simulink model "arducopter"  (R2021a)
settings: Solver=FixedStepAuto  StartTime=0.0  StopTime=sim.param.timeEnd  FixedStep=sim.param.dt  RelTol=1e-3
undefined symbols (not defined in the file or in its folder): DiscIntNeverNeededParam, sim
libraries: simulink x34, slident x4, vrlib x1
(part 2 of 8)

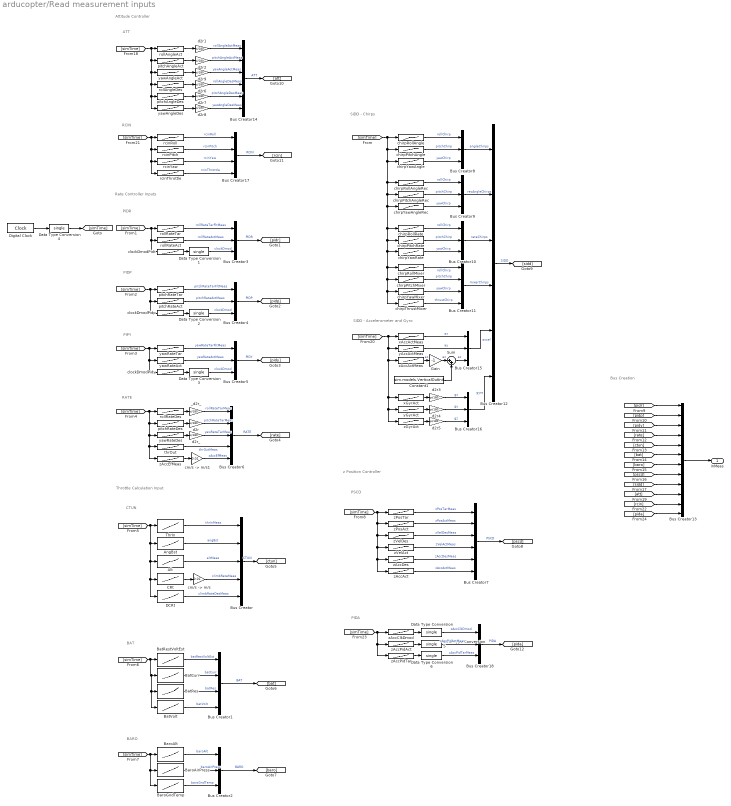
== system arducopter/Read measurement inputs ==
  note: PIDA
  note: Rate Controller Inputs
  note: SIDD - Chirps
  note: PIDR
  note: PIDP
  note: PIPY
  note: RATE
  note: CTUN
  note: BAT
  note: BARO
  note: Throttle Calculation Input
  note: PSCD
  note: z Position Controller
  note: Bus Creation
  note: ATT
  note: Attitude Controller
  note: SIDD - Accelerometer and Gyro
  note: RCIN
  Alt : Lookup_n-D  NumberOfTableDimensions=1  BreakpointsForDimension1=sim.signals.CTUN.Time  Table=sim.signals.CTUN.Alt  TableDataTypeStr=single  InternalRulePriority=Speed  OutDataTypeStr=Inherit: Inherit from 'Table data'  RndMeth=Simplest  InputSameDT=on
  AngBst : Lookup_n-D  NumberOfTableDimensions=1  BreakpointsForDimension1=sim.signals.CTUN.Time  Table=sim.signals.CTUN.AngBst  TableDataTypeStr=single  InternalRulePriority=Speed  OutDataTypeStr=Inherit: Inherit from 'Table data'  RndMeth=Simplest  InputSameDT=on
  BaroAirPress : Lookup_n-D  NumberOfTableDimensions=1  BreakpointsForDimension1=sim.signals.BARO.Time  Table=sim.signals.BARO.AirPress  TableDataTypeStr=Inherit: Inherit from 'Table data'  InternalRulePriority=Speed  OutDataTypeStr=Inherit: Inherit from 'Table data'  RndMeth=Simplest  InputSameDT=on
  BaroAlt : Lookup_n-D  NumberOfTableDimensions=1  BreakpointsForDimension1=sim.signals.BARO.Time  Table=sim.signals.BARO.Alt  TableDataTypeStr=Inherit: Inherit from 'Table data'  InternalRulePriority=Speed  OutDataTypeStr=Inherit: Inherit from 'Table data'  RndMeth=Simplest  InputSameDT=on
  BaroGndTemp : Lookup_n-D  NumberOfTableDimensions=1  BreakpointsForDimension1=sim.signals.BARO.Time  Table=sim.signals.BARO.GndTemp  TableDataTypeStr=Inherit: Inherit from 'Table data'  InternalRulePriority=Speed  OutDataTypeStr=Inherit: Inherit from 'Table data'  RndMeth=Simplest  InputSameDT=on
  BatCurr : Lookup_n-D  NumberOfTableDimensions=1  BreakpointsForDimension1=sim.signals.BAT.Time  Table=sim.signals.BAT.Curr  TableDataTypeStr=single  InternalRulePriority=Speed  OutDataTypeStr=Inherit: Inherit from 'Table data'  RndMeth=Simplest  InputSameDT=on
  BatRes : Lookup_n-D  NumberOfTableDimensions=1  BreakpointsForDimension1=sim.signals.BAT.Time  Table=sim.signals.BAT.Res  TableDataTypeStr=single  InternalRulePriority=Speed  OutDataTypeStr=Inherit: Inherit from 'Table data'  RndMeth=Simplest  InputSameDT=on
  BatRestVoltEst : Lookup_n-D  NumberOfTableDimensions=1  BreakpointsForDimension1=sim.signals.BAT.Time  Table=sim.signals.BAT.RestVoltEst  TableDataTypeStr=single  InternalRulePriority=Speed  OutDataTypeStr=Inherit: Inherit from 'Table data'  RndMeth=Simplest  InputSameDT=on
  BatVolt : Lookup_n-D  NumberOfTableDimensions=1  BreakpointsForDimension1=sim.signals.BAT.Time  Table=sim.signals.BAT.Volt  TableDataTypeStr=Inherit: Inherit from 'Table data'  InternalRulePriority=Speed  OutDataTypeStr=Inherit: Inherit from 'Table data'  RndMeth=Simplest  InputSameDT=on
  Bus Creator : BusCreator  Inputs=5
  Bus Creator1 : BusCreator  Inputs=4
  Bus Creator{2..5,8..10,15..16,18} (10 alike) : BusCreator  Inputs=3
  Bus Creator11 : BusCreator  Inputs=4
  Bus Creator12 : BusCreator  Inputs=6
  Bus Creator13 : BusCreator  Inputs=12
  Bus Creator14 : BusCreator  Inputs=6
  Bus Creator17 : BusCreator  Inputs=4
  Bus Creator6 : BusCreator  Inputs=5
  Bus Creator7 : BusCreator  Inputs=6
  CRt : Lookup_n-D  NumberOfTableDimensions=1  BreakpointsForDimension1=sim.signals.CTUN.Time  Table=sim.signals.CTUN.CRt  TableDataTypeStr=single  InternalRulePriority=Speed  OutDataTypeStr=Inherit: Inherit from 'Table data'  RndMeth=Simplest  InputSameDT=on
  Constant1 : Constant  Value=sim.models.VerticalOutInit
  DCRt : Lookup_n-D  NumberOfTableDimensions=1  BreakpointsForDimension1=sim.signals.CTUN.Time  Table=sim.signals.CTUN.DCRt  TableDataTypeStr=single  InternalRulePriority=Speed  OutDataTypeStr=Inherit: Inherit from 'Table data'  RndMeth=Simplest  InputSameDT=on
  Data Type Conversion{,1..6} (7 alike) : DataTypeConversion  OutDataTypeStr=single
  Digital Clock : DigitalClock  SampleTime=sim.param.dt
  Gain : Gain  Gain=-1
  Sum : Sum  Inputs=|++
  ThrIn : Lookup_n-D  NumberOfTableDimensions=1  BreakpointsForDimension1=sim.signals.CTUN.Time  Table=sim.signals.CTUN.ThrIn  TableDataTypeStr=single  InternalRulePriority=Speed  OutDataTypeStr=Inherit: Inherit from 'Table data'  RndMeth=Simplest  InputSameDT=on
  _d2r_ : Gain  Gain=pi/180
  chirpPitchAngle : Lookup_n-D  NumberOfTableDimensions=1  BreakpointsForDimension1=sim.signals.SIDD.Time{2}  Table=sim.signals.SIDD.Chirp{2}  TableDataTypeStr=Inherit: Inherit from 'Table data'  InternalRulePriority=Speed  OutDataTypeStr=Inherit: Inherit from 'Table data'  RndMeth=Simplest  InputSameDT=on
  chirpPitchAngleRec : Lookup_n-D  NumberOfTableDimensions=1  BreakpointsForDimension1=sim.signals.SIDD.Time{5}  Table=sim.signals.SIDD.Chirp{5}  TableDataTypeStr=Inherit: Inherit from 'Table data'  InternalRulePriority=Speed  OutDataTypeStr=Inherit: Inherit from 'Table data'  RndMeth=Simplest  InputSameDT=on
  chirpPitchMixer : Lookup_n-D  NumberOfTableDimensions=1  BreakpointsForDimension1=sim.signals.SIDD.Time{11}  Table=sim.signals.SIDD.Chirp{11}  TableDataTypeStr=Inherit: Inherit from 'Table data'  InternalRulePriority=Speed  OutDataTypeStr=Inherit: Inherit from 'Table data'  RndMeth=Simplest  InputSameDT=on
  chirpPitchRate : Lookup_n-D  NumberOfTableDimensions=1  BreakpointsForDimension1=sim.signals.SIDD.Time{8}  Table=sim.signals.SIDD.Chirp{8}  TableDataTypeStr=Inherit: Inherit from 'Table data'  InternalRulePriority=Speed  OutDataTypeStr=Inherit: Inherit from 'Table data'  RndMeth=Simplest  InputSameDT=on
  chirpRollAngle : Lookup_n-D  NumberOfTableDimensions=1  BreakpointsForDimension1=sim.signals.SIDD.Time{1}  Table=sim.signals.SIDD.Chirp{1}  TableDataTypeStr=Inherit: Inherit from 'Table data'  InternalRulePriority=Speed  OutDataTypeStr=Inherit: Inherit from 'Table data'  RndMeth=Simplest  InputSameDT=on
  chirpRollAngleRec : Lookup_n-D  NumberOfTableDimensions=1  BreakpointsForDimension1=sim.signals.SIDD.Time{4}  Table=sim.signals.SIDD.Chirp{4}  TableDataTypeStr=Inherit: Inherit from 'Table data'  InternalRulePriority=Speed  OutDataTypeStr=Inherit: Inherit from 'Table data'  RndMeth=Simplest  InputSameDT=on
  chirpRollMixer : Lookup_n-D  NumberOfTableDimensions=1  BreakpointsForDimension1=sim.signals.SIDD.Time{10}  Table=sim.signals.SIDD.Chirp{10}  TableDataTypeStr=Inherit: Inherit from 'Table data'  InternalRulePriority=Speed  OutDataTypeStr=Inherit: Inherit from 'Table data'  RndMeth=Simplest  InputSameDT=on
  chirpRollRate : Lookup_n-D  NumberOfTableDimensions=1  BreakpointsForDimension1=sim.signals.SIDD.Time{7}  Table=sim.signals.SIDD.Chirp{7}  TableDataTypeStr=Inherit: Inherit from 'Table data'  InternalRulePriority=Speed  OutDataTypeStr=Inherit: Inherit from 'Table data'  RndMeth=Simplest  InputSameDT=on
  chirpThrustMixer : Lookup_n-D  NumberOfTableDimensions=1  BreakpointsForDimension1=sim.signals.SIDD.Time{13}  Table=sim.signals.SIDD.Chirp{13}  TableDataTypeStr=Inherit: Inherit from 'Table data'  InternalRulePriority=Speed  OutDataTypeStr=Inherit: Inherit from 'Table data'  RndMeth=Simplest  InputSameDT=on
  chirpYawAngle : Lookup_n-D  NumberOfTableDimensions=1  BreakpointsForDimension1=sim.signals.SIDD.Time{3}  Table=sim.signals.SIDD.Chirp{3}  TableDataTypeStr=Inherit: Inherit from 'Table data'  InternalRulePriority=Speed  OutDataTypeStr=Inherit: Inherit from 'Table data'  RndMeth=Simplest  InputSameDT=on
  chirpYawAngleRec : Lookup_n-D  NumberOfTableDimensions=1  BreakpointsForDimension1=sim.signals.SIDD.Time{6}  Table=sim.signals.SIDD.Chirp{6}  TableDataTypeStr=Inherit: Inherit from 'Table data'  InternalRulePriority=Speed  OutDataTypeStr=Inherit: Inherit from 'Table data'  RndMeth=Simplest  InputSameDT=on
  chirpYawMixer : Lookup_n-D  NumberOfTableDimensions=1  BreakpointsForDimension1=sim.signals.SIDD.Time{12}  Table=sim.signals.SIDD.Chirp{12}  TableDataTypeStr=Inherit: Inherit from 'Table data'  InternalRulePriority=Speed  OutDataTypeStr=Inherit: Inherit from 'Table data'  RndMeth=Simplest  InputSameDT=on
  chirpYawRate : Lookup_n-D  NumberOfTableDimensions=1  BreakpointsForDimension1=sim.signals.SIDD.Time{9}  Table=sim.signals.SIDD.Chirp{9}  TableDataTypeStr=Inherit: Inherit from 'Table data'  InternalRulePriority=Speed  OutDataTypeStr=Inherit: Inherit from 'Table data'  RndMeth=Simplest  InputSameDT=on
  clockDmodPidp : Lookup_n-D  NumberOfTableDimensions=1  BreakpointsForDimension1=sim.signals.PIDP.Time  Table=sim.signals.PIDP.ClockDMod  InternalRulePriority=Speed  RndMeth=Simplest  InputSameDT=on
  clockDmodPidr : Lookup_n-D  NumberOfTableDimensions=1  BreakpointsForDimension1=sim.signals.PIDR.Time  Table=sim.signals.PIDR.ClockDMod  TableDataTypeStr=Inherit: Inherit from 'Table data'  InternalRulePriority=Speed  OutDataTypeStr=Inherit: Inherit from 'Table data'  RndMeth=Simplest  InputSameDT=on
  clockDmodPidy : Lookup_n-D  NumberOfTableDimensions=1  BreakpointsForDimension1=sim.signals.PIDY.Time  Table=sim.signals.PIDY.ClockDMod  InternalRulePriority=Speed  RndMeth=Simplest  InputSameDT=on
  "cm/s -> m/s" : Gain  Gain=0.01
  "cm/s -> m/s1" : Gain  Gain=0.01
  d2r{,1..9} (10 alike) : Gain  Gain=pi/180
  d2r_ : Gain  Gain=pi/180
  pitchAngleAct : Lookup_n-D  NumberOfTableDimensions=1  BreakpointsForDimension1=sim.signals.ATT.Time  Table=sim.signals.ATT.Pitch  TableDataTypeStr=Inherit: Inherit from 'Table data'  InternalRulePriority=Speed  OutDataTypeStr=Inherit: Inherit from 'Table data'  RndMeth=Simplest  InputSameDT=on
  pitchAngleDes : Lookup_n-D  NumberOfTableDimensions=1  BreakpointsForDimension1=sim.signals.ATT.Time  Table=sim.signals.ATT.DesPitch  TableDataTypeStr=Inherit: Inherit from 'Table data'  InternalRulePriority=Speed  OutDataTypeStr=Inherit: Inherit from 'Table data'  RndMeth=Simplest  InputSameDT=on
  pitchRateAct : Lookup_n-D  NumberOfTableDimensions=1  BreakpointsForDimension1=sim.signals.PIDP.Time  Table=sim.signals.PIDP.Act  TableDataTypeStr=Inherit: Inherit from 'Table data'  InternalRulePriority=Speed  OutDataTypeStr=Inherit: Inherit from 'Table data'  RndMeth=Simplest  InputSameDT=on
  pitchRateDes : Lookup_n-D  NumberOfTableDimensions=1  BreakpointsForDimension1=sim.signals.RATE.Time  Table=sim.signals.RATE.PDes  TableDataTypeStr=Inherit: Inherit from 'Table data'  InternalRulePriority=Speed  OutDataTypeStr=Inherit: Inherit from 'Table data'  RndMeth=Simplest  InputSameDT=on
  pitchRateTar : Lookup_n-D  NumberOfTableDimensions=1  BreakpointsForDimension1=sim.signals.PIDP.Time  Table=sim.signals.PIDP.Tar  TableDataTypeStr=Inherit: Inherit from 'Table data'  InternalRulePriority=Speed  OutDataTypeStr=Inherit: Inherit from 'Table data'  RndMeth=Simplest  InputSameDT=on
  rcinPitch : Lookup_n-D  NumberOfTableDimensions=1  BreakpointsForDimension1=sim.signals.RCIN.Time  Table=sim.signals.RCIN.PitchInput  InterpMethod=Linear Lagrange  ExtrapMethod=Clip  InternalRulePriority=Speed  OutDataTypeStr=Inherit: Inherit from 'Table data'  RndMeth=Simplest  InputSameDT=on
  rcinRoll : Lookup_n-D  NumberOfTableDimensions=1  BreakpointsForDimension1=sim.signals.RCIN.Time  Table=sim.signals.RCIN.RollInput  TableDataTypeStr=Inherit: Inherit from 'Table data'  ExtrapMethod=Clip  InternalRulePriority=Speed  OutDataTypeStr=Inherit: Inherit from 'Table data'  RndMeth=Simplest  InputSameDT=on
  rcinThrottle : Lookup_n-D  NumberOfTableDimensions=1  BreakpointsForDimension1=sim.signals.RCIN.Time  Table=sim.signals.RCIN.ThrottleInput  TableDataTypeStr=Inherit: Inherit from 'Table data'  ExtrapMethod=Clip  InternalRulePriority=Speed  OutDataTypeStr=Inherit: Inherit from 'Table data'  RndMeth=Simplest  InputSameDT=on
  rcinYaw : Lookup_n-D  NumberOfTableDimensions=1  BreakpointsForDimension1=sim.signals.RCIN.Time  Table=sim.signals.RCIN.YawInput  TableDataTypeStr=Inherit: Inherit from 'Table data'  ExtrapMethod=Clip  InternalRulePriority=Speed  OutDataTypeStr=Inherit: Inherit from 'Table data'  RndMeth=Simplest  InputSameDT=on
  rollAngleAct : Lookup_n-D  NumberOfTableDimensions=1  BreakpointsForDimension1=sim.signals.ATT.Time  Table=sim.signals.ATT.Roll  TableDataTypeStr=Inherit: Inherit from 'Table data'  InternalRulePriority=Speed  OutDataTypeStr=Inherit: Inherit from 'Table data'  RndMeth=Simplest  InputSameDT=on
  rollAngleDes : Lookup_n-D  NumberOfTableDimensions=1  BreakpointsForDimension1=sim.signals.ATT.Time  Table=sim.signals.ATT.DesRoll  TableDataTypeStr=Inherit: Inherit from 'Table data'  InternalRulePriority=Speed  OutDataTypeStr=Inherit: Inherit from 'Table data'  RndMeth=Simplest  InputSameDT=on
  rollRateAct : Lookup_n-D  NumberOfTableDimensions=1  BreakpointsForDimension1=sim.signals.PIDR.Time  Table=sim.signals.PIDR.Act  TableDataTypeStr=Inherit: Inherit from 'Table data'  InternalRulePriority=Speed  OutDataTypeStr=Inherit: Inherit from 'Table data'  RndMeth=Simplest  InputSameDT=on
  rollRateDes : Lookup_n-D  NumberOfTableDimensions=1  BreakpointsForDimension1=sim.signals.RATE.Time  Table=sim.signals.RATE.RDes  TableDataTypeStr=Inherit: Inherit from 'Table data'  InternalRulePriority=Speed  OutDataTypeStr=Inherit: Inherit from 'Table data'  RndMeth=Simplest  InputSameDT=on
  rollRateTar : Lookup_n-D  NumberOfTableDimensions=1  BreakpointsForDimension1=sim.signals.PIDR.Time  Table=sim.signals.PIDR.Tar  TableDataTypeStr=Inherit: Inherit from 'Table data'  InternalRulePriority=Speed  OutDataTypeStr=Inherit: Inherit from 'Table data'  RndMeth=Simplest  InputSameDT=on
  thrOut : Lookup_n-D  NumberOfTableDimensions=1  BreakpointsForDimension1=sim.signals.RATE.Time  Table=sim.signals.RATE.AOut  TableDataTypeStr=Inherit: Inherit from 'Table data'  InternalRulePriority=Speed  OutDataTypeStr=Inherit: Inherit from 'Table data'  RndMeth=Simplest  InputSameDT=on
  xAccActMeas : Lookup_n-D  NumberOfTableDimensions=1  BreakpointsForDimension1=sim.signals.SIDD.Time{1}  Table=sim.signals.SIDD.AccX  TableDataTypeStr=Inherit: Inherit from 'Table data'  InternalRulePriority=Speed  OutDataTypeStr=Inherit: Inherit from 'Table data'  RndMeth=Simplest  InputSameDT=on
  xGyrAct : Lookup_n-D  NumberOfTableDimensions=1  BreakpointsForDimension1=sim.signals.SIDD.Time{1}  Table=sim.signals.SIDD.GyrX  TableDataTypeStr=Inherit: Inherit from 'Table data'  InternalRulePriority=Speed  OutDataTypeStr=Inherit: Inherit from 'Table data'  RndMeth=Simplest  InputSameDT=on
  yAccActMeas : Lookup_n-D  NumberOfTableDimensions=1  BreakpointsForDimension1=sim.signals.SIDD.Time{1}  Table=sim.signals.SIDD.AccY  TableDataTypeStr=Inherit: Inherit from 'Table data'  InternalRulePriority=Speed  OutDataTypeStr=Inherit: Inherit from 'Table data'  RndMeth=Simplest  InputSameDT=on
  yGyrAct : Lookup_n-D  NumberOfTableDimensions=1  BreakpointsForDimension1=sim.signals.SIDD.Time{1}  Table=sim.signals.SIDD.GyrY  TableDataTypeStr=Inherit: Inherit from 'Table data'  InternalRulePriority=Speed  OutDataTypeStr=Inherit: Inherit from 'Table data'  RndMeth=Simplest  InputSameDT=on
  yawAngleAct : Lookup_n-D  NumberOfTableDimensions=1  BreakpointsForDimension1=sim.signals.ATT.Time  Table=sim.signals.ATT.Yaw  TableDataTypeStr=Inherit: Inherit from 'Table data'  InternalRulePriority=Speed  OutDataTypeStr=Inherit: Inherit from 'Table data'  RndMeth=Simplest  InputSameDT=on
  yawAngleDes : Lookup_n-D  NumberOfTableDimensions=1  BreakpointsForDimension1=sim.signals.ATT.Time  Table=sim.signals.ATT.DesYaw  TableDataTypeStr=Inherit: Inherit from 'Table data'  InternalRulePriority=Speed  OutDataTypeStr=Inherit: Inherit from 'Table data'  RndMeth=Simplest  InputSameDT=on
  yawRateAct : Lookup_n-D  NumberOfTableDimensions=1  BreakpointsForDimension1=sim.signals.PIDY.Time  Table=sim.signals.PIDY.Act  TableDataTypeStr=Inherit: Inherit from 'Table data'  InternalRulePriority=Speed  OutDataTypeStr=Inherit: Inherit from 'Table data'  RndMeth=Simplest  InputSameDT=on
  yawRateDes : Lookup_n-D  NumberOfTableDimensions=1  BreakpointsForDimension1=sim.signals.RATE.Time  Table=sim.signals.RATE.YDes  TableDataTypeStr=Inherit: Inherit from 'Table data'  InternalRulePriority=Speed  OutDataTypeStr=Inherit: Inherit from 'Table data'  RndMeth=Simplest  InputSameDT=on
  yawRateTar : Lookup_n-D  NumberOfTableDimensions=1  BreakpointsForDimension1=sim.signals.PIDY.Time  Table=sim.signals.PIDY.Tar  TableDataTypeStr=Inherit: Inherit from 'Table data'  InternalRulePriority=Speed  OutDataTypeStr=Inherit: Inherit from 'Table data'  RndMeth=Simplest  InputSameDT=on
  zAccAct : Lookup_n-D  NumberOfTableDimensions=1  BreakpointsForDimension1=sim.signals.PSCD.Time  Table=sim.signals.PSCD.zAccAct  TableDataTypeStr=single  InternalRulePriority=Speed  OutDataTypeStr=Inherit: Inherit from 'Table data'  RndMeth=Simplest  InputSameDT=on
  zAccActMeas : Lookup_n-D  NumberOfTableDimensions=1  BreakpointsForDimension1=sim.signals.SIDD.Time{1}  Table=sim.signals.SIDD.AccZ  TableDataTypeStr=Inherit: Inherit from 'Table data'  InternalRulePriority=Speed  OutDataTypeStr=Inherit: Inherit from 'Table data'  RndMeth=Simplest  InputSameDT=on
  zAccClkDmod : Lookup_n-D  NumberOfTableDimensions=1  BreakpointsForDimension1=sim.signals.PIDA.Time  Table=sim.signals.PIDA.ClockDMod  InternalRulePriority=Speed  RndMeth=Simplest  InputSameDT=on
  zAccDes : Lookup_n-D  NumberOfTableDimensions=1  BreakpointsForDimension1=sim.signals.PSCD.Time  Table=sim.signals.PSCD.zAccDes  TableDataTypeStr=single  InternalRulePriority=Speed  OutDataTypeStr=Inherit: Inherit from 'Table data'  RndMeth=Simplest  InputSameDT=on
  zAccEfMeas : Lookup_n-D  NumberOfTableDimensions=1  BreakpointsForDimension1=sim.signals.RATE.Time  Table=sim.signals.RATE.A  TableDataTypeStr=Inherit: Inherit from 'Table data'  InternalRulePriority=Speed  OutDataTypeStr=Inherit: Inherit from 'Table data'  RndMeth=Simplest  InputSameDT=on
  zAccPidAct : Lookup_n-D  NumberOfTableDimensions=1  BreakpointsForDimension1=sim.signals.PIDA.Time  Table=sim.signals.PIDA.Act  InternalRulePriority=Speed  RndMeth=Simplest  InputSameDT=on
  zAccPidTar : Lookup_n-D  NumberOfTableDimensions=1  BreakpointsForDimension1=sim.signals.PIDA.Time  Table=sim.signals.PIDA.Tar  InternalRulePriority=Speed  RndMeth=Simplest  InputSameDT=on
  zGyrAct : Lookup_n-D  NumberOfTableDimensions=1  BreakpointsForDimension1=sim.signals.SIDD.Time{1}  Table=sim.signals.SIDD.GyrZ  TableDataTypeStr=Inherit: Inherit from 'Table data'  InternalRulePriority=Speed  OutDataTypeStr=Inherit: Inherit from 'Table data'  RndMeth=Simplest  InputSameDT=on
  zPosAct : Lookup_n-D  NumberOfTableDimensions=1  BreakpointsForDimension1=sim.signals.PSCD.Time  Table=sim.signals.PSCD.zPosAct  TableDataTypeStr=single  InternalRulePriority=Speed  OutDataTypeStr=Inherit: Inherit from 'Table data'  RndMeth=Simplest  InputSameDT=on
  zPosTar : Lookup_n-D  NumberOfTableDimensions=1  BreakpointsForDimension1=sim.signals.PSCD.Time  Table=sim.signals.PSCD.zPosTar  TableDataTypeStr=single  InternalRulePriority=Speed  OutDataTypeStr=Inherit: Inherit from 'Table data'  RndMeth=Simplest  InputSameDT=on
  zVelAct : Lookup_n-D  NumberOfTableDimensions=1  BreakpointsForDimension1=sim.signals.PSCD.Time  Table=sim.signals.PSCD.zVelAct  TableDataTypeStr=Inherit: Inherit from 'Table data'  InternalRulePriority=Speed  OutDataTypeStr=single  RndMeth=Simplest  InputSameDT=on
  zVelDes : Lookup_n-D  NumberOfTableDimensions=1  BreakpointsForDimension1=sim.signals.PSCD.Time  Table=sim.signals.PSCD.zVelDes  TableDataTypeStr=single  InternalRulePriority=Speed  OutDataTypeStr=Inherit: Inherit from 'Table data'  RndMeth=Simplest  InputSameDT=on
  inMeas : Outport
  wires:
  Digital Clock/1 -> Data Type Conversion4/1
  [simTime] -> chirpThrustMixer/1, chirpYawMixer/1, chirpPitchMixer/1, chirpRollMixer/1, chirpYawRate/1, chirpPitchRate/1, chirpRollRate/1, chirpYawAngleRec/1, chirpPitchAngleRec/1, chirpRollAngleRec/1, chirpYawAngle/1, chirpPitchAngle/1, chirpRollAngle/1
  [simTime] -> clockDmodPidr/1, rollRateAct/1, rollRateTar/1
  [simTime] -> clockDmodPidp/1, pitchRateAct/1, pitchRateTar/1
  [simTime] -> yawRateAct/1, clockDmodPidy/1, yawRateTar/1
  [simTime] -> rollRateDes/1, zAccEfMeas/1, thrOut/1, yawRateDes/1, pitchRateDes/1
  ThrIn/1 -> Bus Creator/1  "thrInMeas"
  BaroAlt/1 -> Bus Creator2/1  "baroAlt"
  BaroAirPress/1 -> Bus Creator2/2  "baroAirPress"
  AngBst/1 -> Bus Creator/2  "angBst"
  BatCurr/1 -> Bus Creator1/2  "batCurr"
  BatVolt/1 -> Bus Creator1/4  "batVolt"
  BaroGndTemp/1 -> Bus Creator2/3  "baroGndTemp"
  BatRes/1 -> Bus Creator1/3  "batRes"
  BatRestVoltEst/1 -> Bus Creator1/1  "batRestVoltEst"
  [simTime] -> CRt/1, DCRt/1, Alt/1, AngBst/1, ThrIn/1
  [simTime] -> BatVolt/1, BatRes/1, BatCurr/1, BatRestVoltEst/1
  [simTime] -> BaroGndTemp/1, BaroAirPress/1, BaroAlt/1
  rollRateTar/1 -> Bus Creator3/1  "rollRateTarFltMeas"
  clockDmodPidr/1 -> Data Type Conversion1/1
  pitchRateTar/1 -> Bus Creator4/1  "pitchRateTarFltMeas"
  clockDmodPidp/1 -> Data Type Conversion2/1
  yawRateAct/1 -> Bus Creator5/2  "yawRateActMeas"
  yawRateTar/1 -> Bus Creator5/1  "yawRateTarFltMeas"
  clockDmodPidy/1 -> Data Type Conversion3/1
  pitchRateDes/1 -> d2r/1
  rollRateDes/1 -> _d2r_/1
  yawRateDes/1 -> d2r_/1
  d2r_/1 -> Bus Creator6/3  "yawRateTarMeas"
  Bus Creator3/1 -> [pidr]  "PIDR"
  Bus Creator4/1 -> [pidp]  "PIDP"
  Bus Creator5/1 -> [pidy]  "PIDY"
  Bus Creator6/1 -> [rate]  "RATE"
  Bus Creator/1 -> [ctun]  "CTUN"
  Bus Creator1/1 -> [bat]  "BAT"
  Bus Creator2/1 -> [baro]  "BARO"
  zPosAct/1 -> Bus Creator7/2  "zPosActMeas"
  zVelDes/1 -> Bus Creator7/3  "zVelDesMeas"
  zVelAct/1 -> Bus Creator7/4  "zVelActMeas"
  zAccAct/1 -> Bus Creator7/6  "zAccActMeas"
  zPosTar/1 -> Bus Creator7/1  "zPosTarMeas"
  zAccDes/1 -> Bus Creator7/5  "zAccDesMeas"
  [simTime] -> zPosAct/1, zAccAct/1, zAccDes/1, zVelAct/1, zVelDes/1, zPosTar/1
  Bus Creator7/1 -> [pscd]  "PSCD"
  Data Type Conversion1/1 -> Bus Creator3/3  "clockDmod"
  Data Type Conversion2/1 -> Bus Creator4/3  "clockDmod"
  Data Type Conversion3/1 -> Bus Creator5/3  "clockDmod"
  chirpPitchAngle/1 -> Bus Creator8/2  "pitchChirp"
  chirpRollAngle/1 -> Bus Creator8/1  "rollChirp"
  chirpYawAngle/1 -> Bus Creator8/3  "yawChirp"
  Bus Creator8/1 -> Bus Creator12/1  "angleChirps"
  chirpPitchAngleRec/1 -> Bus Creator9/2  "pitchChirp"
  chirpRollAngleRec/1 -> Bus Creator9/1  "rollChirp"
  chirpYawAngleRec/1 -> Bus Creator9/3  "yawChirp"
  Bus Creator9/1 -> Bus Creator12/2  "recAngleChirps"
  chirpPitchRate/1 -> Bus Creator10/2  "pitchChirp"
  chirpRollRate/1 -> Bus Creator10/1  "rollChirp"
  chirpYawRate/1 -> Bus Creator10/3  "yawChirp"
  Bus Creator10/1 -> Bus Creator12/3  "rateChirps"
  chirpRollMixer/1 -> Bus Creator11/1  "rollChirp"
  chirpPitchMixer/1 -> Bus Creator11/2  "pitchChirp"
  chirpYawMixer/1 -> Bus Creator11/3  "yawChirp"
  Bus Creator11/1 -> Bus Creator12/4  "mixerChirps"
  chirpThrustMixer/1 -> Bus Creator11/4  "thrustChirp"
  Bus Creator12/1 -> [sidd]  "SIDD"
  Bus Creator13/1 -> inMeas/1
  [pidr] -> Bus Creator13/1
  [pidp] -> Bus Creator13/2
  [pidy] -> Bus Creator13/3
  [rate] -> Bus Creator13/4
  [ctun] -> Bus Creator13/5
  [bat] -> Bus Creator13/6
  [baro] -> Bus Creator13/7
  [pscd] -> Bus Creator13/8
  [sidd] -> Bus Creator13/9
  Data Type Conversion4/1 -> [simTime]
  pitchRateAct/1 -> Bus Creator4/2  "pitchRateActMeas"
  _d2r_/1 -> Bus Creator6/1  "rollRateTarMeas"
  rollRateAct/1 -> Bus Creator3/2  "rollRateActMeas"
  d2r/1 -> Bus Creator6/2  "pitchRateTarMeas"
  d2r2/1 -> Bus Creator14/2  "pitchAngleActMeas"
  Bus Creator14/1 -> [att]  "ATT"
  d2r1/1 -> Bus Creator14/1  "rollAngleActMeas"
  [simTime] -> rollAngleAct/1, yawAngleAct/1, yawAngleDes/1, pitchAngleDes/1, rollAngleDes/1, pitchAngleAct/1
  [att] -> Bus Creator13/10
  [simTime] -> zGyrAct/1, yGyrAct/1, xGyrAct/1, zAccActMeas/1, yAccActMeas/1, xAccActMeas/1
  xAccActMeas/1 -> Bus Creator15/1  "ax"
  yAccActMeas/1 -> Bus Creator15/2  "ay"
  xGyrAct/1 -> d2r3/1
  yGyrAct/1 -> d2r4/1
  zGyrAct/1 -> d2r5/1
  Bus Creator15/1 -> Bus Creator12/5  "accel"
  Bus Creator16/1 -> Bus Creator12/6  "gyro"
  rollAngleAct/1 -> d2r1/1
  pitchAngleAct/1 -> d2r2/1
  d2r3/1 -> Bus Creator16/1  "gx"
  d2r4/1 -> Bus Creator16/2  "gy"
  d2r5/1 -> Bus Creator16/3  "gz"
  pitchAngleDes/1 -> d2r7/1
  rollAngleDes/1 -> d2r6/1
  d2r6/1 -> Bus Creator14/4  "rollAngleDesMeas"
  d2r7/1 -> Bus Creator14/5  "pitchAngleDesMeas"
  yawAngleDes/1 -> d2r8/1
  d2r8/1 -> Bus Creator14/6  "yawAngleDesMeas"
  yawAngleAct/1 -> d2r9/1
  d2r9/1 -> Bus Creator14/3  "yawAngleActMeas"
  rcinRoll/1 -> Bus Creator17/1  "rcinRoll"
  rcinPitch/1 -> Bus Creator17/2  "rcinPitch"
  rcinYaw/1 -> Bus Creator17/3  "rcinYaw"
  Bus Creator17/1 -> [rcin]  "RCIN"
  [rcin] -> Bus Creator13/11
  [simTime] -> rcinRoll/1, rcinThrottle/1, rcinYaw/1, rcinPitch/1
  thrOut/1 -> Bus Creator6/4  "thrOutMeas"
  zAccEfMeas/1 -> "cm/s -> m/s1"/1
  zAccActMeas/1 -> Gain/1  "az"
  Alt/1 -> Bus Creator/3  "altMeas"
  CRt/1 -> "cm/s -> m/s"/1
  "cm/s -> m/s"/1 -> Bus Creator/4  "climbRateMeas"
  Sum/1 -> Bus Creator15/3  "az"
  "cm/s -> m/s1"/1 -> Bus Creator6/5  "zAccEfMeas"
  Gain/1 -> Sum/1  "az"
  Constant1/1 -> Sum/2
  Data Type Conversion/1 -> Bus Creator18/1  "zAccClkDmod"
  zAccClkDmod/1 -> Data Type Conversion/1
  [simTime] -> zAccPidTar/1, zAccPidAct/1, zAccClkDmod/1
  zAccPidAct/1 -> Data Type Conversion5/1
  zAccPidTar/1 -> Data Type Conversion6/1
  Data Type Conversion5/1 -> Bus Creator18/2  "zAccPidActMeas"
  Data Type Conversion6/1 -> Bus Creator18/3  "zAccPidTarMeas"
  Bus Creator18/1 -> [pida]  "PIDA"
  [pida] -> Bus Creator13/12
  DCRt/1 -> Bus Creator/5  "climbRateDesMeas"
  rcinThrottle/1 -> Bus Creator17/4  "rcinThrottle"

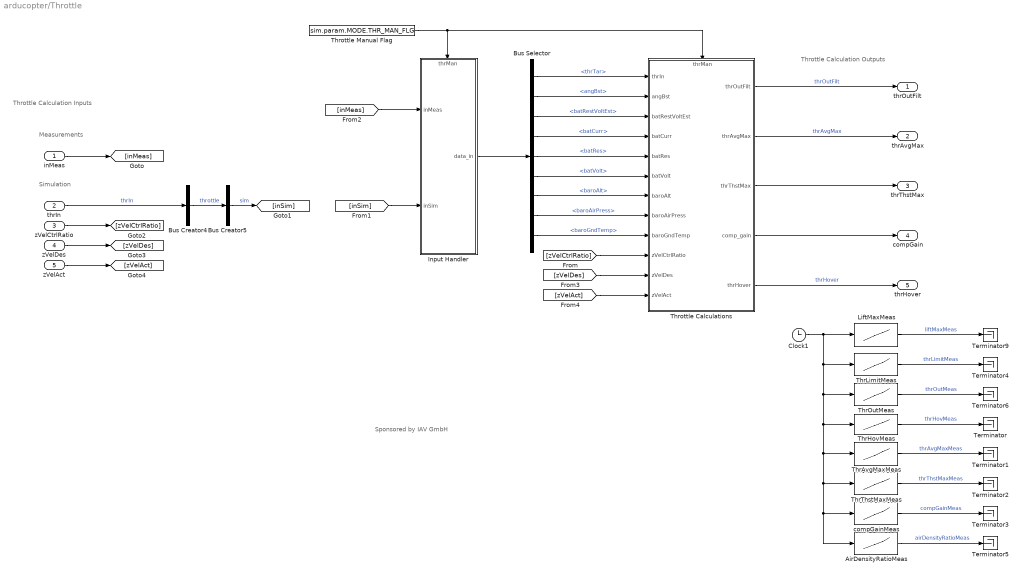
== system arducopter/Throttle ==
  note: Throttle Calculation Outputs
  note: Throttle Calculation Inputs
  note: Simulation
  note: Measurements
  note: Sponsored by IAV GmbH
  inMeas : Inport
  thrIn : Inport  Port=2
  zVelCtrlRatio : Inport  Port=3
  zVelDes : Inport  Port=4
  zVelAct : Inport  Port=5
  AirDensityRatioMeas : Lookup_n-D  NumberOfTableDimensions=1  BreakpointsForDimension1=sim.signals.MOTQ.Time  Table=sim.signals.MOTQ.CompGain  InternalRulePriority=Speed  RndMeth=Simplest  InputSameDT=on
  Bus Creator4 : BusCreator  Inputs=1
  Bus Creator5 : BusCreator  Inputs=1
  Bus Selector : BusSelector  OutputSignals=thrTar,angBst,batRestVoltEst,batCurr,batRes,batVolt,baroAlt,baroAirPress,baroGndTemp
  Clock1 : Clock
  Input Handler : Subsystem
  LiftMaxMeas : Lookup_n-D  NumberOfTableDimensions=1  BreakpointsForDimension1=sim.signals.MOTB.Time  Table=sim.signals.MOTB.LiftMax  InternalRulePriority=Speed  RndMeth=Simplest  InputSameDT=on
  Terminator{,1..6,9} (8 alike) : Terminator
  ThrAvgMaxMeas : Lookup_n-D  NumberOfTableDimensions=1  BreakpointsForDimension1=sim.signals.MOTB.Time  Table=sim.signals.MOTB.ThrAvMx  InternalRulePriority=Speed  RndMeth=Simplest  InputSameDT=on
  ThrHovMeas : Lookup_n-D  NumberOfTableDimensions=1  BreakpointsForDimension1=sim.signals.CTUN.Time  Table=sim.signals.CTUN.ThrHov  InternalRulePriority=Speed  RndMeth=Simplest  InputSameDT=on
  ThrLimitMeas : Lookup_n-D  NumberOfTableDimensions=1  BreakpointsForDimension1=sim.signals.MOTB.Time  Table=sim.signals.MOTB.ThrLimit  InternalRulePriority=Speed  RndMeth=Simplest  InputSameDT=on
  ThrOutMeas : Lookup_n-D  NumberOfTableDimensions=1  BreakpointsForDimension1=sim.signals.CTUN.Time  Table=sim.signals.CTUN.ThrOut  InternalRulePriority=Speed  RndMeth=Simplest  InputSameDT=on
  ThrThstMaxMeas : Lookup_n-D  NumberOfTableDimensions=1  BreakpointsForDimension1=sim.signals.MOTQ.Time  Table=sim.signals.MOTQ.ThrThstMaxMeas  InternalRulePriority=Speed  RndMeth=Simplest  InputSameDT=on
  Throttle Calculations : Subsystem
  Throttle Manual Flag : Constant  Value=sim.param.MODE.THR_MAN_FLG
  compGainMeas : Lookup_n-D  NumberOfTableDimensions=1  BreakpointsForDimension1=sim.signals.MOTQ.Time  Table=sim.signals.MOTQ.CompGain  InternalRulePriority=Speed  RndMeth=Simplest  InputSameDT=on
  thrOutFilt : Outport
  thrAvgMax : Outport  Port=2
  thrThstMax : Outport  Port=3
  compGain : Outport  Port=4
  thrHover : Outport  Port=5
  wires:
  Bus Selector/4 -> Throttle Calculations/4(batCurr)  "<batCurr>"
  Throttle Calculations/2(thrAvgMax) -> thrAvgMax/1  "thrAvgMax"
  Bus Selector/8 -> Throttle Calculations/8(baroAirPress)  "<baroAirPress>"
  Bus Selector/6 -> Throttle Calculations/6(batVolt)  "<batVolt>"
  Throttle Calculations/1(thrOutFilt) -> thrOutFilt/1  "thrOutFilt"
  Bus Selector/2 -> Throttle Calculations/2(angBst)  "<angBst>"
  Bus Selector/1 -> Throttle Calculations/1(thrIn)  "<thrTar>"
  Bus Selector/7 -> Throttle Calculations/7(baroAlt)  "<baroAlt>"
  Bus Selector/3 -> Throttle Calculations/3(batRestVoltEst)  "<batRestVoltEst>"
  Bus Selector/5 -> Throttle Calculations/5(batRes)  "<batRes>"
  Throttle Calculations/3(thrThstMax) -> thrThstMax/1
  Throttle Calculations/4(comp_gain) -> compGain/1
  Throttle Calculations/5(thrHover) -> thrHover/1  "thrHover"
  thrIn/1 -> Bus Creator4/1  "thrIn"
  Bus Creator4/1 -> Bus Creator5/1  "throttle"
  Bus Creator5/1 -> [inSim]  "sim"
  [inSim] -> Input Handler/2(inSim)
  [inMeas] -> Input Handler/1(inMeas)
  Throttle Manual Flag/1 -> Throttle Calculations/13(thrMan), Input Handler/3(thrMan)
  Input Handler/1(data_in) -> Bus Selector/1
  Bus Selector/9 -> Throttle Calculations/9(baroGndTemp)  "<baroGndTemp>"
  ThrHovMeas/1 -> Terminator/1  "thrHovMeas"
  LiftMaxMeas/1 -> Terminator9/1  "liftMaxMeas"
  ThrOutMeas/1 -> Terminator6/1  "thrOutMeas"
  ThrLimitMeas/1 -> Terminator4/1  "thrLimitMeas"
  zVelCtrlRatio/1 -> [zVelCtrlRatio]
  [zVelCtrlRatio] -> Throttle Calculations/10(zVelCtrlRatio)
  zVelDes/1 -> [zVelDes]
  [zVelDes] -> Throttle Calculations/11(zVelDes)
  [zVelAct] -> Throttle Calculations/12(zVelAct)
  zVelAct/1 -> [zVelAct]
  ThrAvgMaxMeas/1 -> Terminator1/1  "thrAvgMaxMeas"
  ThrThstMaxMeas/1 -> Terminator2/1  "thrThstMaxMeas"
  compGainMeas/1 -> Terminator3/1  "compGainMeas"
  AirDensityRatioMeas/1 -> Terminator5/1  "airDensityRatioMeas"
  Clock1/1 -> ThrLimitMeas/1, ThrHovMeas/1, AirDensityRatioMeas/1, compGainMeas/1, ThrThstMaxMeas/1, ThrAvgMaxMeas/1, ThrOutMeas/1, LiftMaxMeas/1
  inMeas/1 -> [inMeas]

== system arducopter/radioIn to controlIn ==
  note: high_in = 1000, defined in Copter::init_rc_in()
  note: Calculation of control values from radio input.
      | The functions are called from pwm_to_range() or pwm_to_ange() (roll,pitch,yaw) in RC_Channel::update().
      | For the throttle channel, the pwm_to_range() function is called, since it is a range type radio channel (Copter::default_dead_zones() -> channel_throttle->set_range())
  note: norm_input_dz() in control.cpp
      | Called in ModeStabilize::run() to norm the yaw radio input of the pilot
  note: Sponsored by IAV GmbH
  rcInRoll : Inport
  rcInPitch : Inport  Port=2
  rcInYaw : Inport  Port=3
  rcInThrottle : Inport  Port=4
  Constant : Constant  Value=sim.param.RCIN.DZ_RLL
  Constant1 : Constant  Value=sim.param.RCIN.MIN_RLL
  Constant10 : Constant  Value=sim.param.RCIN.DZ_YAW
  Constant11 : Constant  Value=sim.param.RCIN.MIN_YAW
  Constant12 : Constant  Value=sim.param.RCIN.MAX_YAW
  Constant13 : Constant  Value=sim.param.RCIN.REVERSED_YAW
  Constant15 : Constant  Value=sim.param.RCIN.TRIM_PIT
  Constant16 : Constant  Value=sim.param.RCIN.TRIM_YAW
  Constant17 : Constant  Value=sim.param.RCIN.TRIM_RLL
  Constant18 : Constant  Value=sim.param.RCIN.DZ_THR
  Constant19 : Constant  Value=sim.param.RCIN.MIN_THR
  Constant2 : Constant  Value=sim.param.RCIN.MAX_RLL
  Constant20 : Constant  Value=sim.param.RCIN.MAX_THR
  Constant21 : Constant  Value=sim.param.RCIN.REVERSED_THR
  Constant22 : Constant  Value=1000
  Constant3 : Constant  Value=sim.param.RCIN.REVERSED_RLL
  Constant4 : Constant  Value=sim.param.RCIN.ROLL_PITCH_YAW_INPUT_MAX
  Constant5 : Constant  Value=sim.param.RCIN.DZ_PIT
  Constant6 : Constant  Value=sim.param.RCIN.MIN_PIT
  Constant7 : Constant  Value=sim.param.RCIN.MAX_PIT
  Constant8 : Constant  Value=sim.param.RCIN.REVERSED_PIT
  Constant9 : Constant  Value=sim.param.RCIN.ROLL_PITCH_YAW_INPUT_MAX
  MATLAB Function : MATLAB Function  TreatAsAtomicUnit=on
  MATLAB Function1 : MATLAB Function  TreatAsAtomicUnit=on
  MATLAB Function2 : MATLAB Function  TreatAsAtomicUnit=on
  MATLAB Function3 : MATLAB Function  TreatAsAtomicUnit=on
  ctrlInRoll : Outport
  ctrlInPitch : Outport  Port=2
  ctrlInYaw : Outport  Port=3
  ctrlInThrottle : Outport  Port=4
  wires:
  rcInRoll/1 -> MATLAB Function/1(rcIn)
  Constant/1 -> MATLAB Function/2(deadZone)
  Constant1/1 -> MATLAB Function/3(radioMin)
  Constant2/1 -> MATLAB Function/4(radioMax)
  Constant3/1 -> MATLAB Function/6(reversed)
  Constant4/1 -> MATLAB Function/7(highIn)
  Constant8/1 -> MATLAB Function3/6(reversed)
  Constant9/1 -> MATLAB Function3/7(highIn)
  Constant5/1 -> MATLAB Function3/2(deadZone)
  Constant6/1 -> MATLAB Function3/3(radioMin)
  Constant7/1 -> MATLAB Function3/4(radioMax)
  rcInPitch/1 -> MATLAB Function3/1(rcIn)
  rcInYaw/1 -> MATLAB Function1/1(radioIn)
  MATLAB Function/1(angleIn) -> ctrlInRoll/1
  MATLAB Function3/1(angleIn) -> ctrlInPitch/1
  MATLAB Function1/1(out) -> ctrlInYaw/1
  Constant17/1 -> MATLAB Function/5(trim)
  Constant15/1 -> MATLAB Function3/5(trim)
  MATLAB Function2/1(ctrlIn) -> ctrlInThrottle/1
  rcInThrottle/1 -> MATLAB Function2/1(rcIn)
  Constant21/1 -> MATLAB Function2/5(reversed)
  Constant19/1 -> MATLAB Function2/3(radioMin)
  Constant20/1 -> MATLAB Function2/4(radioMax)
  Constant22/1 -> MATLAB Function2/6(highIn)
  Constant18/1 -> MATLAB Function2/2(deadZone)
  Constant12/1 -> MATLAB Function1/5(radioMax)
  Constant13/1 -> MATLAB Function1/6(reversed)
  Constant10/1 -> MATLAB Function1/2(deadZone)
  Constant16/1 -> MATLAB Function1/3(radioTrim)
  Constant11/1 -> MATLAB Function1/4(radioMin)

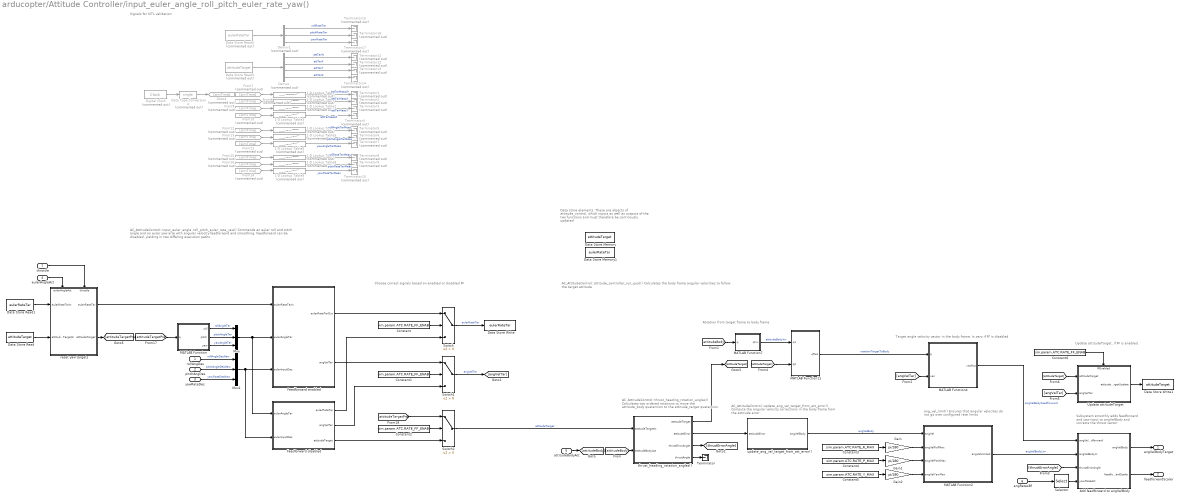
== system arducopter/Attitude Controller/input_euler_angle_roll_pitch_euler_rate_yaw() ==
  note: Signals for SITL validation
  note: Data store elements. These are objects of attitude_control, which inputs as well as outputs of the two functions and must therefore be continously updated
  note: Update attitudeTarget, if FF is enabled.
  note: Subsystem smoothly adds feedforward and yaw input to angVelBody and corrects the thrust vector
  note: Target angle velocity vector in the body frame. Is zero if FF is disabled
  note: Rotation from target frame to body frame
  note: Choose correct signals based on enabled or disabled FF
  note: AC_AttitudeControl::input_euler_angle_roll_pitch_euler_rate_yaw()
      | Commands an euler roll and pitch angle and an euler yaw arte with angular velocity feedforward and smoothing.
      | Feedforward can be disabled, yielding in two differing execution paths.
  note: AC_AttitudeControl::thrust_heading_rotation_angles()
      | Calculates two ordered rotations to move the attitude_body quaternion to the attitude_target quaternion.
  note: AC_AttitudeControl::update_ang_vel_target_from_att_error()
      | Compute the angular velocity corrections in the body frame from the attitude error.
  note: ang_vel_limit()
      | Ensures that angular velocites do not go over configured rate limits
  note: AC_AttitudeControl::attitude_controller_run_quat()
      | Calculates the body frame angular velocities to follow the target attitude
  rollAngDes : Inport
  pitchAngDes : Inport  Port=2
  yawRateDes : Inport  Port=3
  eulerAngleAct : Inport  Port=4
  attitudeBodyAct : Inport  Port=5
  angRatesBf : Inport  Port=6
  throttle : Inport  Port=7
  1-D Lookup Table : Lookup_n-D  Commented=on  NumberOfTableDimensions=1  BreakpointsForDimension1=sim.signals.ATT.Time  Table=sim.signals.ATT.attTarMeasW  InternalRulePriority=Speed  RndMeth=Simplest  InputSameDT=on
  1-D Lookup Table1 : Lookup_n-D  Commented=on  NumberOfTableDimensions=1  BreakpointsForDimension1=sim.signals.ATT.Time  Table=sim.signals.ATT.attTarMeasX  InternalRulePriority=Speed  RndMeth=Simplest  InputSameDT=on
  1-D Lookup Table2 : Lookup_n-D  Commented=on  NumberOfTableDimensions=1  BreakpointsForDimension1=sim.signals.ATT.Time  Table=sim.signals.ATT.attTarMeasY  InternalRulePriority=Speed  RndMeth=Simplest  InputSameDT=on
  1-D Lookup Table3 : Lookup_n-D  Commented=on  NumberOfTableDimensions=1  BreakpointsForDimension1=sim.signals.ATT.Time  Table=sim.signals.ATT.attTarMeasZ  InternalRulePriority=Speed  RndMeth=Simplest  InputSameDT=on
  1-D Lookup Table4 : Lookup_n-D  Commented=on  NumberOfTableDimensions=1  BreakpointsForDimension1=sim.signals.ATT.Time  Table=sim.signals.ATT.eulerAngTarMeasX  InternalRulePriority=Speed  RndMeth=Simplest  InputSameDT=on
  1-D Lookup Table5 : Lookup_n-D  Commented=on  NumberOfTableDimensions=1  BreakpointsForDimension1=sim.signals.ATT.Time  Table=sim.signals.ATT.eulerAngTarMeasY  InternalRulePriority=Speed  RndMeth=Simplest  InputSameDT=on
  1-D Lookup Table6 : Lookup_n-D  Commented=on  NumberOfTableDimensions=1  BreakpointsForDimension1=sim.signals.ATT.Time  Table=sim.signals.ATT.eulerAngTarMeasZ  InternalRulePriority=Speed  RndMeth=Simplest  InputSameDT=on
  1-D Lookup Table7 : Lookup_n-D  Commented=on  NumberOfTableDimensions=1  BreakpointsForDimension1=sim.signals.ATT.Time  Table=sim.signals.ATT.eulerRatTarMeasX  InternalRulePriority=Speed  RndMeth=Simplest  InputSameDT=on
  1-D Lookup Table8 : Lookup_n-D  Commented=on  NumberOfTableDimensions=1  BreakpointsForDimension1=sim.signals.ATT.Time  Table=sim.signals.ATT.eulerRatTarMeasY  InternalRulePriority=Speed  RndMeth=Simplest  InputSameDT=on
  1-D Lookup Table9 : Lookup_n-D  Commented=on  NumberOfTableDimensions=1  BreakpointsForDimension1=sim.signals.ATT.Time  Table=sim.signals.ATT.eulerRatTarMeasZ  InternalRulePriority=Speed  RndMeth=Simplest  InputSameDT=on
  Add feedforward to angVelBody : Subsystem
  Constant{,1..2,6} (4 alike) : Constant  Value=sim.param.ATC.RATE_FF_ENAB
  Constant3 : Constant  Value=sim.param.ATC.RATE_R_MAX
  Constant4 : Constant  Value=sim.param.ATC.RATE_P_MAX
  Constant5 : Constant  Value=sim.param.ATC.RATE_Y_MAX
  Data Store Memory : DataStoreMemory  DataStoreName=attitudeTarget  ReadBeforeWriteMsg=warning  WriteAfterWriteMsg=warning  WriteAfterReadMsg=warning  InitialValue=sim.init.ATT.attitudeTarget  ShowAdditionalParam=off  OutDataTypeStr=single
  Data Store Memory1 : DataStoreMemory  DataStoreName=eulerRateTar  ReadBeforeWriteMsg=warning  WriteAfterWriteMsg=warning  WriteAfterReadMsg=warning  InitialValue=sim.init.ATT.eulerRateTar  ShowAdditionalParam=off  OutDataTypeStr=single
  Data Store Read : DataStoreRead  DataStoreName=attitudeTarget  IndexOptions=Index vector (dialog)  Indices=1  OutputSizes=1
  Data Store Read1 : DataStoreRead  DataStoreName=eulerRateTar  IndexOptions=Index vector (dialog)  Indices=1  OutputSizes=1
  Data Store Read3 : DataStoreRead  Commented=on  DataStoreName=attitudeTarget  IndexOptions=Index vector (dialog)  Indices=1  OutputSizes=1
  Data Store Read4 : DataStoreRead  Commented=on  DataStoreName=eulerRateTar  IndexOptions=Index vector (dialog)  Indices=1  OutputSizes=1
  Data Store Write : DataStoreWrite  DataStoreName=eulerRateTar  IndexOptions=Index vector (dialog)  Indices=1  OutputSizes=1
  Data Store Write1 : DataStoreWrite  DataStoreName=attitudeTarget  IndexOptions=Index vector (dialog)  Indices=1  OutputSizes=1
  Data Type Conversion4 : DataTypeConversion  Commented=on  OutDataTypeStr=single
  Demux : Demux  Commented=on
  Demux1 : Demux  Commented=on  Outputs=3
  Digital Clock : DigitalClock  Commented=on  SampleTime=sim.param.dt
  Feedforward disabled : Subsystem
  Feedforward enabled : Subsystem
  From{7..16} (10 alike) : From  Commented=on  GotoTag=simTime
  Gain : Gain  Gain=pi/180
  Gain1 : Gain  Gain=pi/180
  Gain2 : Gain  Gain=pi/180
  Goto4 : Goto  Commented=on  GotoTag=simTime
  MATLAB Function : MATLAB Function  TreatAsAtomicUnit=on
  MATLAB Function11 : MATLAB Function  TreatAsAtomicUnit=on
  MATLAB Function2 : MATLAB Function  TreatAsAtomicUnit=on
  MATLAB Function4 : MATLAB Function  TreatAsAtomicUnit=on
  MATLAB Function7 : MATLAB Function  TreatAsAtomicUnit=on
  Mux : Mux  Inputs=3
  Mux1 : Mux  Inputs=3
  Selector : Selector  InputPortWidth=3  IndexOptions=Index vector (dialog)  Indices=[3]  OutputSizes=1
  Switch : Switch  Criteria=u2 > Threshold
  Switch1 : Switch  Criteria=u2 > Threshold
  Switch2 : Switch  Criteria=u2 > Threshold
  Terminator : Terminator
  Terminator{1..17} (17 alike) : Terminator  Commented=on
  Update attitudeTarget : Subsystem
  reset yaw targets : Subsystem
  thrust_heading_rotation_angles() : Subsystem
  update_ang_vel_target_from_att_error() : Subsystem
  angVelBodyTarget : Outport
  feedforwardScaler : Outport  Port=2
  wires:
  MATLAB Function/3(yaw) -> Mux/3  "yawAngleTar"
  MATLAB Function/2(pitch) -> Mux/2  "pitchAngleTar"
  MATLAB Function/1(roll) -> Mux/1  "rollAngleTar"
  Mux/1 -> Feedforward disabled/1(eulerAngleTar), Feedforward enabled/2(eulerAngleTar)
  rollAngDes/1 -> Mux1/1  "rollAngleDesNew"
  pitchAngDes/1 -> Mux1/2  "pitchAngleDesNew"
  yawRateDes/1 -> Mux1/3  "yawRateDesNew"
  Mux1/1 -> Feedforward enabled/3(eulerInputDes), Feedforward disabled/2(eulerInputDes)
  Data Store Read1/1 -> reset yaw targets/1(eulerRateTarIn)
  Feedforward enabled/1(eulerRateTarOut) -> Switch/1
  Feedforward disabled/1(eulerRateTar) -> Switch/3
  Feedforward enabled/2(angVelTar) -> Switch1/1
  Constant/1 -> Switch/2
  Feedforward disabled/2(angVelTar) -> Switch1/3
  Switch/1 -> Data Store Write/1  "eulerRateTar"
  Switch1/1 -> [angVelTar]  "angVelTar"
  Constant1/1 -> Switch1/2
  Constant2/1 -> Switch2/2
  [attitudeTargetPre] -> Switch2/1
  Feedforward disabled/3(attitudeTarget) -> Switch2/3
  Switch2/1 -> thrust_heading_rotation_angles()/1(attitudeTargetIn)  "attitudeTarget"
  [attitudeBody] -> thrust_heading_rotation_angles()/2(attitudeBodyAct)
  thrust_heading_rotation_angles()/4(thrustAngle) -> Terminator/1
  thrust_heading_rotation_angles()/2(attitudeError) -> update_ang_vel_target_from_att_error()/1(attitudeError)
  Constant4/1 -> Gain1/1
  Constant3/1 -> Gain/1
  Gain2/1 -> MATLAB Function2/4(angVelYawMax)
  Gain1/1 -> MATLAB Function2/3(angVelPitchMax)
  Constant5/1 -> Gain2/1
  Gain/1 -> MATLAB Function2/2(angVelRollMax)
  update_ang_vel_target_from_att_error()/1(angVelBody) -> MATLAB Function2/1(angVel)  "angVelBody"
  attitudeBodyAct/1 -> [attitudeBody]
  thrust_heading_rotation_angles()/1(attitudeTarget) -> [attitudeTarget]
  [attitudeBody] -> MATLAB Function7/1(q)
  MATLAB Function7/1(qInv) -> MATLAB Function11/1(q1)  "attitudeBodyInv"
  MATLAB Function11/1(qRes) -> MATLAB Function4/1(q)  "rotationTargetToBody"
  [angVelTar] -> MATLAB Function4/2(vec)
  MATLAB Function4/1(vecRot) -> Add feedforward to angVelBody/1(angVelBodyFeedforward)  "angVelBodyFeedforward"
  thrust_heading_rotation_angles()/3(thrustErrorAngle) -> [thrustErrorAngle]
  MATLAB Function2/1(angVelLimited) -> Add feedforward to angVelBody/2(angVelBodyIn)  "angVelBodyLim"
  [thrustErrorAngle] -> Add feedforward to angVelBody/3(thurstErrorAngle)
  angRatesBf/1 -> Selector/1
  Selector/1 -> Add feedforward to angVelBody/4(yawRateAct)
  [attitudeTarget] -> MATLAB Function11/2(q2)
  [angVelTar] -> Update attitudeTarget/2(angVelTar)
  Add feedforward to angVelBody/1(angVelBody) -> angVelBodyTarget/1
  [attitudeTarget] -> Update attitudeTarget/1(attitudeTarget)
  Update attitudeTarget/1(attitudeTargetUpdate) -> Data Store Write1/1
  Constant6/1 -> Update attitudeTarget/3(ffEnabled)
  Add feedforward to angVelBody/2(feedforwardScaler) -> feedforwardScaler/1
  Data Type Conversion4/1 -> Goto4/1
  Digital Clock/1 -> Data Type Conversion4/1
  From7/1 -> 1-D Lookup Table/1
  From8/1 -> 1-D Lookup Table1/1
  From9/1 -> 1-D Lookup Table2/1
  From10/1 -> 1-D Lookup Table3/1
  From11/1 -> 1-D Lookup Table6/1
  From13/1 -> 1-D Lookup Table5/1
  From12/1 -> 1-D Lookup Table4/1
  From15/1 -> 1-D Lookup Table7/1
  From16/1 -> 1-D Lookup Table8/1
  From14/1 -> 1-D Lookup Table9/1
  1-D Lookup Table/1 -> Terminator1/1  "attTarMeasW"
  1-D Lookup Table1/1 -> Terminator2/1  "attTarMeasX"
  1-D Lookup Table2/1 -> Terminator3/1  "attTarMeasY"
  1-D Lookup Table3/1 -> Terminator4/1  "attTarMeasZ"
  1-D Lookup Table6/1 -> Terminator7/1  "yawAngleTarMeas"
  1-D Lookup Table5/1 -> Terminator6/1  "pitchAngleTarMeas"
  1-D Lookup Table4/1 -> Terminator5/1  "rollAngleTarMeas"
  1-D Lookup Table7/1 -> Terminator8/1  "rollRateTarMeas"
  1-D Lookup Table8/1 -> Terminator9/1  "pitchRateTarMeas"
  1-D Lookup Table9/1 -> Terminator10/1  "yawRateTarMeas"
  Data Store Read3/1 -> Demux/1
  Demux/4 -> Terminator14/1  "attTarZ"
  Demux/3 -> Terminator13/1  "attTarY"
  Demux/2 -> Terminator12/1  "attTarX"
  Demux/1 -> Terminator11/1  "attTarW"
  Data Store Read4/1 -> Demux1/1
  Demux1/1 -> Terminator15/1  "rollRateTar"
  Demux1/2 -> Terminator16/1  "pitchRateTar"
  Demux1/3 -> Terminator17/1  "yawRateTar"
  Data Store Read/1 -> reset yaw targets/2(attitudeTargetIn)
  reset yaw targets/1(eulerRateTar) -> Feedforward enabled/1(eulerRateTarIn)
  eulerAngleAct/1 -> reset yaw targets/3(eulerAngleAct)
  [attitudeTargetPre] -> MATLAB Function/1(q)
  reset yaw targets/2(attitudeTarget) -> [attitudeTargetPre]
  throttle/1 -> reset yaw targets/4(throttle)

== system arducopter/Lowpass2p/Lowpass Pitch ==
  u : Inport
  sampleFreq : Inport  Port=2
  cutoffFreq : Inport  Port=3
  Data Store Memory1 : DataStoreMemory  DataStoreName=delElem2  ReadBeforeWriteMsg=warning  WriteAfterWriteMsg=warning  WriteAfterReadMsg=warning  ShowAdditionalParam=off  OutDataTypeStr=single
  Data Store Memory10 : DataStoreMemory  DataStoreName=delElem1  ReadBeforeWriteMsg=warning  WriteAfterWriteMsg=warning  WriteAfterReadMsg=warning  ShowAdditionalParam=off  OutDataTypeStr=single
  Lowpass2p : MATLAB Function  TreatAsAtomicUnit=on
  y : Outport
  wires:
  u/1 -> Lowpass2p/1(u)
  cutoffFreq/1 -> Lowpass2p/3(cutoffFreq)
  sampleFreq/1 -> Lowpass2p/2(sampleFreq)
  Lowpass2p/1(y) -> y/1

== system arducopter/Lowpass2p/Lowpass Roll ==
  u : Inport
  sampleFreq : Inport  Port=2
  cutoffFreq : Inport  Port=3
  Data Store Memory1 : DataStoreMemory  DataStoreName=delElem2  ReadBeforeWriteMsg=warning  WriteAfterWriteMsg=warning  WriteAfterReadMsg=warning  ShowAdditionalParam=off  OutDataTypeStr=single
  Data Store Memory10 : DataStoreMemory  DataStoreName=delElem1  ReadBeforeWriteMsg=warning  WriteAfterWriteMsg=warning  WriteAfterReadMsg=warning  ShowAdditionalParam=off  OutDataTypeStr=single
  Lowpass2p : MATLAB Function  TreatAsAtomicUnit=on
  y : Outport
  wires:
  Lowpass2p/1(y) -> y/1
  sampleFreq/1 -> Lowpass2p/2(sampleFreq)
  cutoffFreq/1 -> Lowpass2p/3(cutoffFreq)
  u/1 -> Lowpass2p/1(u)

== system arducopter/Lowpass2p/Lowpass Yaw ==
  u : Inport
  sampleFreq : Inport  Port=2
  cutoffFreq : Inport  Port=3
  Data Store Memory1 : DataStoreMemory  DataStoreName=delElem2  ReadBeforeWriteMsg=warning  WriteAfterWriteMsg=warning  WriteAfterReadMsg=warning  ShowAdditionalParam=off  OutDataTypeStr=single
  Data Store Memory10 : DataStoreMemory  DataStoreName=delElem1  ReadBeforeWriteMsg=warning  WriteAfterWriteMsg=warning  WriteAfterReadMsg=warning  ShowAdditionalParam=off  OutDataTypeStr=single
  Lowpass2p : MATLAB Function  TreatAsAtomicUnit=on
  y : Outport
  wires:
  u/1 -> Lowpass2p/1(u)
  cutoffFreq/1 -> Lowpass2p/3(cutoffFreq)
  sampleFreq/1 -> Lowpass2p/2(sampleFreq)
  Lowpass2p/1(y) -> y/1

== system arducopter/Position Controller/P Position z ==
  note: AC_PosControl::update_z_controller() - Position controller
  note: Feed-Forward component
      | update_z_controller()
  note: AC_P_1D::update_all()
      | These two Matlab functions represent the update_all() function of the AC_P_1D class. The function basically consists of two parts, the error
      | calculation with limiting (implemented by calc_err) and the square root controller (implemented by sqrt_controller).
  note: Testrun inputs
  note: Parameter
  note: AC_PosControl::set_correction_speed_accel_z()
  posTar : Inport
  posAct : Inport  Port=2
  velDes : Inport  Port=3
  Calculate error : MATLAB Function  TreatAsAtomicUnit=on
  Constant : Constant  Value=0  OutDataTypeStr=single
  Data Type Conversion : DataTypeConversion  OutDataTypeStr=single
  IC1 : InitialCondition  Value=sim.init.PIDA.posTar
  Product : Product
  Scale Factor Z : Subsystem
  Set vertical speed & acceleration limit : Subsystem
  Square Root Controller : MATLAB Function  TreatAsAtomicUnit=on
  Sum : Sum  Inputs=++|
  dt : Constant  Value=sim.param.dt
  ekf_type : Constant  Value=sim.param.EKF_TYPE
  kp_pos : Constant  Value=sim.param.PSCD.P_POS
  speedDnMax : Constant  Value=sim.param.PSCD.VEL_MAX_DN
  speedUpMax : Constant  Value=sim.param.PSCD.VEL_MAX_UP
  zAccMax : Constant  Value=sim.param.PSCD.ACC_MAX_Z
  velTar : Outport
  posTarUpd : Outport  Port=2
  posErr : Outport  Port=3
  wires:
  speedDnMax/1 -> [dnSpeedMax]
  posAct/1 -> Calculate error/2(act)
  posTar/1 -> IC1/1
  speedUpMax/1 -> [upSpeedMax]
  zAccMax/1 -> [zAccMax]
  kp_pos/1 -> [kpPos]
  [errMin] -> Calculate error/3(err_min)
  [errMax] -> Calculate error/4(err_max)
  [dnSpeedMax] -> Set vertical speed & acceleration limit/1(outMin)
  [upSpeedMax] -> Set vertical speed & acceleration limit/2(outMax)
  [zAccMax] -> Set vertical speed & acceleration limit/3(DoutMax)
  Constant/1 -> Set vertical speed & acceleration limit/4(D2OutMax)
  Set vertical speed & acceleration limit/1(errMin) -> [errMin]
  Set vertical speed & acceleration limit/2(errMax) -> [errMax]
  [error] -> Square Root Controller/1(err)
  Set vertical speed & acceleration limit/3(D1max) -> [D1max]
  [D1max] -> Square Root Controller/3(second_ord_lim)
  [kpPos] -> Square Root Controller/2(p)
  dt/1 -> Data Type Conversion/1
  [dt] -> Square Root Controller/4(dt)
  ekf_type/1 -> [ekfType]
  [ekfType] -> Scale Factor Z/1(ekfType)
  Square Root Controller/1(correction_rate) -> Product/2
  Scale Factor Z/1(scale_z) -> Product/1
  Calculate error/1(tar_new) -> posTarUpd/1
  Product/1 -> Sum/2
  velDes/1 -> Sum/1
  Sum/1 -> velTar/1
  Data Type Conversion/1 -> [dt]
  IC1/1 -> Calculate error/1(tar)
  Calculate error/2(err) -> [error]
  [error] -> posErr/1
  [kpPos] -> Set vertical speed & acceleration limit/5(kp)
